simulink model "Lyp3"  (R2018b)
settings: Solver=FixedStepAuto  StartTime=0.0  StopTime=100  FixedStep=0.001  RelTol=1e-3  EnableMultiTasking=on
InitFcn:
  | X0 = randn(1)*10 ;
settings Model: Creator=omid_zandi  LastModifiedBy=Arash
settings OptimizationCC: LifeSpan=inf
settings DebuggingCC: SFUnexpectedBacktrackingDiag=warning  SFNoUnconditionalDefaultTransitionDiag=warning
settings SFSimCC: SimUseLocalCustomCode=off
settings RTWCC: RTWUseLocalCustomCode=off
settings CodeAppCC: StateflowObjectComments=on
settings GRTTargetCC: TargetLangStandard=C89/C90 (ANSI)  GeneratePreprocessorConditionals=Disable all
settings ConfigComp: CovMetricSettings=dw  CovHtmlReporting=on  CovSaveCumulativeToWorkspaceVar=on  CovSaveSingleToWorkspaceVar=on  CovExternalEMLEnable=off

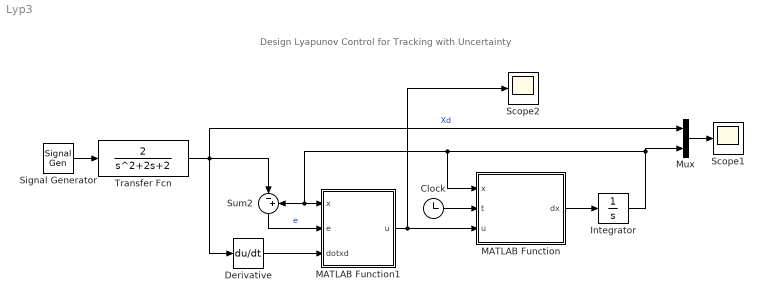
== system Lyp3 ==
  note: Design Lyapunov Control for Tracking with Uncertainty
  Clock : Clock
  Derivative : Derivative
  Integrator : Integrator  InitialCondition=randn
  MATLAB Function : MATLAB Function  TreatAsAtomicUnit=on
  MATLAB Function1 : MATLAB Function  TreatAsAtomicUnit=on
  Mux : Mux  Inputs=2
  Scope1 : Scope
  Scope2 : Scope
  Signal Generator : SignalGenerator  Frequency=0.05
  Sum2 : Sum  Inputs=|-+
  Transfer Fcn : TransferFcn  Numerator=[2]  Denominator=[1 2 2 ]
  wires:
  Signal Generator/1 -> Transfer Fcn/1
  Transfer Fcn/1 -> Mux/1, Sum2/1, Derivative/1  "Xd"
  Derivative/1 -> MATLAB Function1/3(dotxd)
  Sum2/1 -> MATLAB Function1/2(e)  "e"
  MATLAB Function/1(dx) -> Integrator/1
  Integrator/1 -> Mux/2, Sum2/2, MATLAB Function1/1(x), MATLAB Function/1(x)
  Clock/1 -> MATLAB Function/2(t)
  MATLAB Function1/1(u) -> Scope2/1, MATLAB Function/3(u)
  Mux/1 -> Scope1/1

== matlab function Lyp3/MATLAB Function1 ==
  data: x input; u output; e input; dotxd input
function u = fcn(x, e ,dotxd)
F = 2*abs(x) + x^2 + abs(dotxd) ;
u  =  -e - sign(e)*F ;

== matlab function Lyp3/MATLAB Function ==
  data: x input; t input; u input; dx output
function dx = fcn(x, t, u)
a = 1 + sin(2*pi*0.1*t) ; 
b = cos(2*pi*0.1*t) ;
dx = a * x + b * x^2 + u;
